simulink model "Test"  (R2023b)
settings: Solver=VariableStepAuto  StartTime=0.0  StopTime=0.1  RelTol=1e-3
values from neighbouring files (symbols this model uses):
  C_dc = 15e-3    (= 0.015)    [PARAMETERS_MODEL_GR2.m]    (also in Parameters.m; Parameters_Chloe.m)
  f_grid = 50    [PARAMETERS_MODEL_GR2.m]    (also in Parameters.m; Parameters_Chloe.m)
  L_grid = 1.5e-6    (= 1.5e-06)    [PARAMETERS_MODEL_GR2.m]    (also in Parameters.m = 2e-05; Parameters_Chloe.m = 2e-05)
  R_grid = 0.005    [PARAMETERS_MODEL_GR2.m]    (also in Parameters.m = 0.2; Parameters_Chloe.m = 0.2)
  Ts = 5e-6    (= 5e-06)    [PARAMETERS_MODEL_GR2.m]    (also in Parameters.m = 1e-05; Parameters_Chloe.m = 1e-05)
  U_ac = 380    [PARAMETERS_MODEL_GR2.m]    (also in Parameters.m; Parameters_Chloe.m)
libraries: spsDiodeLib x6, spsSeriesRLCBranchLib x4, spsACVoltageSourceLib x3, spsThreePhaseVIMeasurementLib x2, spsGroundLib x1, spsThreePhaseTransformerTwoWindingsLib x1, sps_lib x1
settings Model: Creator=dimit  LastModifiedBy=dimit

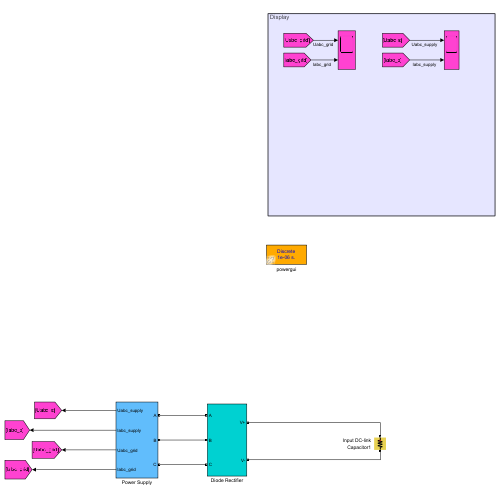
[thumbnail: Simulink's stored preview of the top-level diagram]
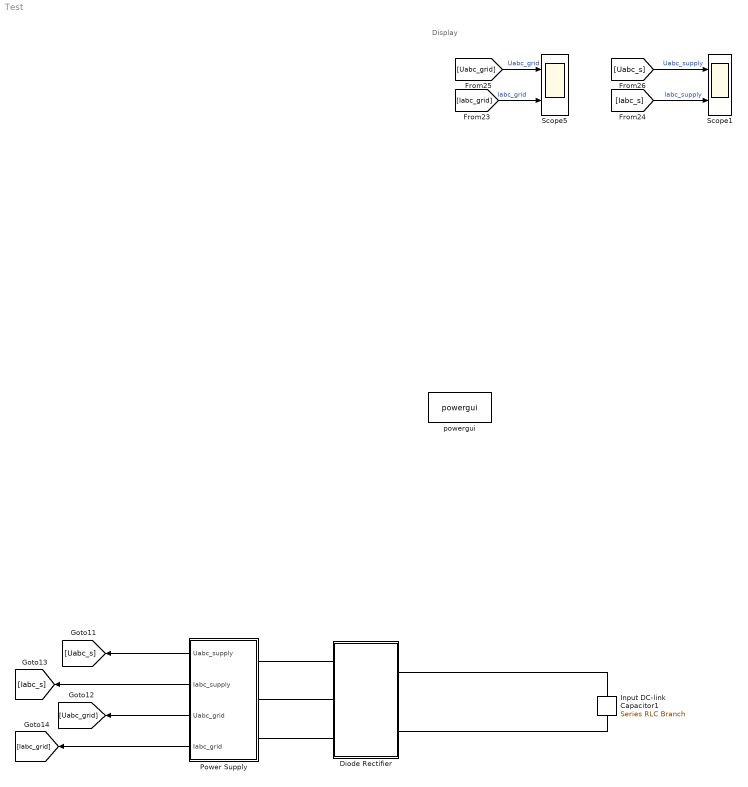
== system Test ==
  note: Display
  Diode Rectifier : Subsystem
  Input DC-link Capacitor1 : spsSeriesRLCBranchLib/Series RLC Branch  LConnTagsString=__new0  RConnTagsString=__new0  BranchType=R  Resistance=20  Inductance=1e-3  SetiL0=off  InitialCurrent=0  Capacitance=C_dc  Setx0=off  InitialVoltage=0  Measurements=None
  Power Supply : Subsystem
  Scope1 : Scope  NumInputPorts=2
  Scope5 : Scope  NumInputPorts=2
  powergui : sps_lib/powergui  Priority=1  SimulationMode=Discrete  SampleTime=Ts  frequency=60  Iterations=50  frequencyindice=50  Pbase=100e6  ErrMax=1e-4  UnitsV=kV  UnitsW=MW  buscounter=0  FunctionMessages=off  echomessages=off  EnableUseOfTLC=off  CurrentSourceSwitches=off  DisableSnubberDevices=off  DisableRonSwitches=off  DisableVfSwitches=off  DisplayEquations=off  AutomaticDiscreteSolvers=off  SolverType=Tustin/Backward Euler (TBE)  Interpol=off  ExternalGateDelay=off  methode=off  Ts=100  x0status=blocks  SPID=on  SwTol=0  HookPort=off  NonlinearTolerance=1e-4  nMaxIteration=100  ContinueOnMaxIteration=off  RestoreLinks=warning  ResistiveCurrentMeasurement=off  Frange=[0:2:500]  Ylog=off  Xlog=on  ShowGrid=off  save=off  variable=ZData  structure=0  ZoomFFT=off  StartTime=0.0  cycles=1  DisplayStyle=1  fundamental=60  FreqAxis=off  MaxFrequency=1000  frequencyindicesteady=1  RmsSteady=1  display=off
  wires:
  [Uabc_grid] -> Scope5/1  "Uabc_grid"
  [Iabc_grid] -> Scope5/2  "Iabc_grid"
  [Iabc_s] -> Scope1/2  "Iabc_supply"
  [Uabc_s] -> Scope1/1  "Uabc_supply"
  Power Supply/2(Iabc_supply) -> [Iabc_s]
  Power Supply/4(Iabc_grid) -> [Iabc_grid]
  Power Supply/1(Uabc_supply) -> [Uabc_s]
  Power Supply/3(Uabc_grid) -> [Uabc_grid]
  connections:
  Diode Rectifier/LConn1 -- Power Supply/LConn1
  Diode Rectifier/LConn2 -- Power Supply/LConn2
  Diode Rectifier/LConn3 -- Power Supply/LConn3
  Input DC-link Capacitor1/RConn1 -- Diode Rectifier/RConn2
  Diode Rectifier/RConn1 -- Input DC-link Capacitor1/LConn1

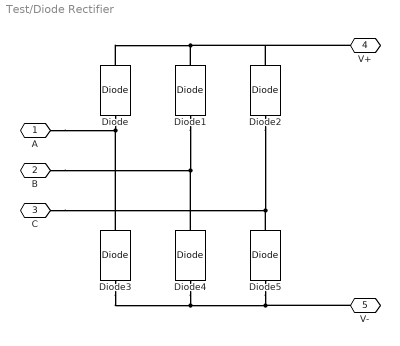
== system Test/Diode Rectifier ==
  Diode{,1..5} (6 alike) : spsDiodeLib/Diode  Ron=R_on_rect  Lon=0  Vf=V_f_rect  IC=0  UseSnubber=0  Rs=R_snub_rect  Cs=C_snub_rect  Measurements=off
  A : PMIOPort  Side=Left
  B : PMIOPort  Port=2  Side=Left
  C : PMIOPort  Port=3  Side=Left
  V+ : PMIOPort  Port=4  Side=Right
  V- : PMIOPort  Port=5  Side=Right
  connections:
  B/RConn1 -- Diode4/RConn1 -- Diode1/LConn1
  Diode4/LConn1 -- Diode3/LConn1 -- Diode5/LConn1 -- V-/RConn1
  C/RConn1 -- Diode5/RConn1 -- Diode2/LConn1
  Diode/LConn1 -- Diode3/RConn1 -- A/RConn1
  Diode/RConn1 -- Diode1/RConn1 -- Diode2/RConn1 -- V+/RConn1

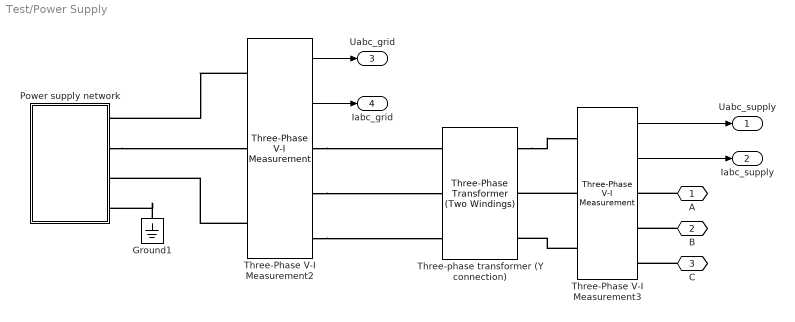
== system Test/Power Supply ==
  Ground1 : spsGroundLib/Ground  LConnTagsString=a
  Power supply network : Subsystem
  Three-Phase V-I Measurement2 : spsThreePhaseVIMeasurementLib/Three-Phase V-I Measurement  VoltageMeasurement=phase-to-phase  SetLabelV=off  LabelV=Vabc  Vpu=off  VpuLL=off  CurrentMeasurement=yes  SetLabelI=off  LabelI=Iabc  Ipu=off  Pbase=100e6  Vbase=500e3  OutputType=Complex  PhasorSimulation=off  PSBequivalent=0
  Three-Phase V-I Measurement3 : spsThreePhaseVIMeasurementLib/Three-Phase V-I Measurement  VoltageMeasurement=phase-to-phase  SetLabelV=off  LabelV=Vabc  Vpu=off  VpuLL=off  CurrentMeasurement=yes  SetLabelI=off  LabelI=Iabc  Ipu=off  Pbase=100e6  Vbase=500e3  OutputType=Complex  PhasorSimulation=off  PSBequivalent=0
  Three-phase transformer (Y connection) : spsThreePhaseTransformerTwoWindingsLib/Three-Phase Transformer (Two Windings)  Winding1Connection=Y  Winding2Connection=Yg  CoreType=Three single-phase transformers  SetSaturation=off  Hysteresis=off  DataFile='hysteresis'  SetInitialFlux=off  Measurements=None  UNITS=pu  NominalPower=[ 20e3 , 50 ]  Winding1=[ 380 , 0.002 , 0.08 ]  Winding2=[ 380 , 0.002 , 80 ]  Rm=500  Lm=500  L0=0.5  Saturation=[ 0,0 ; 0.0024,1.2 ; 1.0,1.52 ]  InitialFluxes=[ 0.8 , -0.8 , 0.7 ]  BreakLoop=off  DiscreteSolver=Trapezoidal iterative  DataType=off  TransfoNumber=1
  A : PMIOPort  Side=Left
  B : PMIOPort  Port=2  Side=Left
  C : PMIOPort  Port=3  Side=Left
  Uabc_supply : Outport  VectorParamsAs1DForOutWhenUnconnected=off
  Iabc_supply : Outport  Port=2  VectorParamsAs1DForOutWhenUnconnected=off
  Uabc_grid : Outport  Port=3  VectorParamsAs1DForOutWhenUnconnected=off
  Iabc_grid : Outport  Port=4  VectorParamsAs1DForOutWhenUnconnected=off
  wires:
  Three-Phase V-I Measurement3/1 -> Uabc_supply/1
  Three-Phase V-I Measurement3/2 -> Iabc_supply/1
  Three-Phase V-I Measurement2/2 -> Iabc_grid/1
  Three-Phase V-I Measurement2/1 -> Uabc_grid/1
  connections:
  Three-Phase V-I Measurement2/LConn3 -- Power supply network/LConn3
  Three-Phase V-I Measurement2/RConn1 -- Three-phase transformer (Y connection)/LConn1
  Power supply network/LConn2 -- Three-Phase V-I Measurement2/LConn2
  Ground1/LConn1 -- Power supply network/LConn4
  Three-Phase V-I Measurement3/LConn2 -- Three-phase transformer (Y connection)/RConn2
  Three-phase transformer (Y connection)/RConn1 -- Three-Phase V-I Measurement3/LConn1
  Three-Phase V-I Measurement2/LConn1 -- Power supply network/LConn1
  Three-Phase V-I Measurement2/RConn2 -- Three-phase transformer (Y connection)/LConn2
  Three-Phase V-I Measurement2/RConn3 -- Three-phase transformer (Y connection)/LConn3
  Three-Phase V-I Measurement3/LConn3 -- Three-phase transformer (Y connection)/RConn3
  C/RConn1 -- Three-Phase V-I Measurement3/RConn3
  A/RConn1 -- Three-Phase V-I Measurement3/RConn1
  B/RConn1 -- Three-Phase V-I Measurement3/RConn2

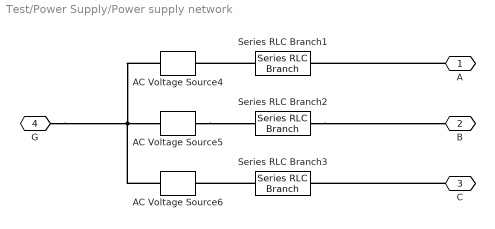
== system Test/Power Supply/Power supply network ==
  AC Voltage Source4 : spsACVoltageSourceLib/AC Voltage Source  Amplitude=U_ac/sqrt(3)*sqrt(2)  Phase=0  Frequency=f_grid  SampleTime=0  Measurements=None  BusType=swing  Pref=10e3  Qref=0  Qmin=-inf  Qmax=+inf
  AC Voltage Source5 : spsACVoltageSourceLib/AC Voltage Source  Amplitude=U_ac/sqrt(3)*sqrt(2)  Phase=-120  Frequency=f_grid  SampleTime=0  Measurements=None  BusType=swing  Pref=10e3  Qref=0  Qmin=-inf  Qmax=+inf
  AC Voltage Source6 : spsACVoltageSourceLib/AC Voltage Source  Amplitude=U_ac/sqrt(3)*sqrt(2)  Phase=120  Frequency=f_grid  SampleTime=0  Measurements=None  BusType=swing  Pref=10e3  Qref=0  Qmin=-inf  Qmax=+inf
  Series RLC Branch1 : spsSeriesRLCBranchLib/Series RLC Branch  LConnTagsString=__new0  RConnTagsString=__new0  BranchType=RL  Resistance=R_grid  Inductance=L_grid  SetiL0=off  InitialCurrent=0  Capacitance=15e-6  Setx0=off  InitialVoltage=0  Measurements=None
  Series RLC Branch2 : spsSeriesRLCBranchLib/Series RLC Branch  LConnTagsString=__new0  RConnTagsString=__new0  BranchType=RL  Resistance=R_grid  Inductance=L_grid  SetiL0=off  InitialCurrent=0  Capacitance=15e-6  Setx0=off  InitialVoltage=0  Measurements=None
  Series RLC Branch3 : spsSeriesRLCBranchLib/Series RLC Branch  LConnTagsString=__new0  RConnTagsString=__new0  BranchType=RL  Resistance=R_grid  Inductance=L_grid  SetiL0=off  InitialCurrent=0  Capacitance=15e-6  Setx0=off  InitialVoltage=0  Measurements=None
  A : PMIOPort  Side=Left
  B : PMIOPort  Port=2  Side=Left
  C : PMIOPort  Port=3  Side=Left
  G : PMIOPort  Port=4  Side=Left
  connections:
  A/RConn1 -- Series RLC Branch1/LConn1
  C/RConn1 -- Series RLC Branch3/LConn1
  AC Voltage Source5/RConn1 -- Series RLC Branch2/RConn1
  Series RLC Branch3/RConn1 -- AC Voltage Source6/RConn1
  Series RLC Branch2/LConn1 -- B/RConn1
  AC Voltage Source6/LConn1 -- G/RConn1 -- AC Voltage Source5/LConn1 -- AC Voltage Source4/LConn1
  Series RLC Branch1/RConn1 -- AC Voltage Source4/RConn1
